simulink model "SF108A_MotCurrPeakEstimn"  (R2013b)
settings: Solver=FixedStepDiscrete  StartTime=0.0  StopTime=1  FixedStep=Ts  RelTol=1e-3
undefined symbols (not defined in the file): ARCHGLBPRM_100MILLISEC_SEC_F32, ARCHGLBPRM_2MILLISEC_SEC_F32
libraries: Fil x6, NxtrLim x2, simulink x1
settings Model: Creator=qzwc4r  LastModifiedBy=BZHF94
settings DataIOCC: LimitDataPoints=off  SaveFormat=Structure  ReturnWorkspaceOutputs=on
settings OptimizationCC: BlockReduction=off  InlineParams=on  ZeroExternalMemoryAtStartup=off  ZeroInternalMemoryAtStartup=off  OptimizeModelRefInitCode=on  LifeSpan=1
settings DebuggingCC: SignalInfNanChecking=error  SignalRangeChecking=warning  UnderspecifiedInitializationDetection=Simplified  SolverPrmCheckMsg=error  InheritedTsInSrcMsg=error  DiscreteInheritContinuousMsg=error  SingleTaskRateTransMsg=error  TasksWithSamePriorityMsg=error  SigSpecEnsureSampleTimeMsg=error  CheckMatrixSingularityMsg=error  IntegerOverflowMsg=error  ParameterUnderflowMsg=error  ParameterPrecisionLossMsg=error  ParameterTunabilityLossMsg=error  FixptConstUnderflowMsg=warning  FixptConstOverflowMsg=warning  VectorMatrixConversionMsg=error  SignalLabelMismatchMsg=error  UnconnectedInputMsg=error  UnconnectedOutputMsg=error  UnconnectedLineMsg=error  SFcnCompatibilityMsg=error  UniqueDataStoreMsg=warning  BusObjectLabelMismatch=error  RootOutportRequireBusObject=error  AssertControl=DisableAll  ModelReferenceIOMsg=error  ModelReferenceVersionMismatchMessage=warning  ModelReferenceIOMismatchMessage=error  ModelReferenceCSMismatchMessage=warning  ModelReferenceDataLoggingMessage=error  StateNameClashWarn=warning  StrictBusMsg=ErrorOnBusTreatedAsVector  NonBusSignalsTreatedAsBus=error  SFUnexpectedBacktrackingDiag=error  SFInvalidInputDataAccessInChartInitDiag=error  SFNoUnconditionalDefaultTransitionDiag=error  SFTransitionOutsideNaturalParentDiag=error  SFUnconditionalTransitionShadowingDiag=error  SFUndirectedBroadcastEventsDiag=error
settings ModelReferenceCC: ModelReferenceNumInstancesAllowed=Single
settings RTWCC: SystemTargetFile=autosar.tlc  GenCodeOnly=on  TemplateMakefile=ert_default_tmf  Description=AUTOSAR  GenerateReport=on  ProcessScript=autosar_make_rtw_hook  LaunchReport=on
settings CodeAppCC: GenerateComments=off  IgnoreCustomStorageClasses=off  CustomSymbolStrType=$N$R$M  CustomSymbolStrBlkIO=$N$M  SimulinkBlockComments=off
settings STFCustomTargetCC: ParMdlRefBuildCompliant=on  CompOptLevelCompliant=on  IncludeMdlTerminateFcn=off  CombineOutputUpdateFcns=on  SuppressErrorStatus=on  ERTFirstTimeCompliant=on  ERTCustomFileBanners=on  SupportNonFinite=off  SupportComplex=off  SupportContinuousTime=off  SupportNonInlinedSFcns=off  MATLABClassNameForMDSCustomization=Simulink.SoftwareTarget.ERTCustomization  AutosarCompliant=on  GRTInterface=off  SystemTargetFile=autosar.tlc
settings ERTTargetCC: CodeReplacementLibrary=ANSI_C  ConcurrentExecutionCompliant=off  IncludeMdlTerminateFcn=off  SuppressErrorStatus=on  SupportNonFinite=off  SupportComplex=off  ModelStepFunctionPrototypeControlCompliant=off  CPPClassGenCompliant=off  AutosarCompliant=on  InlinedParameterPlacement=NonHierarchical  ERTCustomFileTemplate=example_file_process.tlc  EnableUserReplacementTypes=on

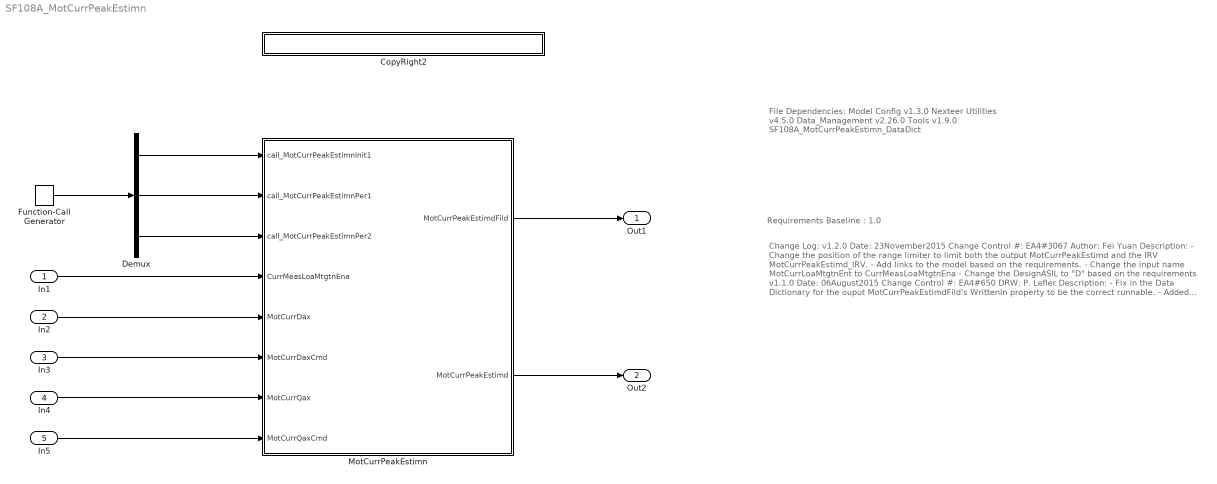
== system SF108A_MotCurrPeakEstimn ==
  note: Requirements Baseline : 1.0
  note: File Dependencies:
      |
      | Model Config v1.3.0
      | Nexteer Utilities v4.5.0
      | Data_Management v2.26.0
      | Tools v1.9.0
      | SF108A_MotCurrPeakEstimn_DataDict
  note: Change Log:
      |
      | v1.2.0
      | Date: 23November2015
      | Change Control #: EA4#3067
      | Author: Fei Yuan
      | Description:
      | - Change the position of the range limiter to limit both the output MotCurrPeakEstimd
      |   and the IRV MotCurrPeakEstimd_IRV.
      | - Add links to the model based on the requirements.
      | - Change the input name MotCurrLoaMtgtnEnt to CurrMeasLoaMtgtnEna
      | - Change the DesignASIL to "D" based on the requirements
      |
      | v1.1.0
      | Date: 06August2015
      | Change Control #: EA4#650
      | DRW: P. Lefler
      | Description:
      | - Fix in the Data Dictionary for the ouput MotCurrPeakEstimdFild's WrittenIn
      |    property to be the correct runnable.
      | - Added range limiters to both of the functions outputs.
      |
      | v1.0.0
      | Date: 17July2015
      | Change Control #: EA4#650
      | DRW: P. Lefler
      | Description:
      | - Initial Release
  In1 : Inport
  In2 : Inport  Port=2
  In3 : Inport  Port=3
  In4 : Inport  Port=4
  In5 : Inport  Port=5
  CopyRight2 : Subsystem  Description=|  mask(Copyright Information){none=on}
      | Copyright info block.                                               
      |                                                                     
      | Place copyright information at the top of every subsystem in design.
      mask prompts: none "No parameters"
      mask help: Place copyright information at the top of every subsystem in design.
      mask Display:
      | NxtrConf = 'Nexteer Confidential';
      | 
      | sys = bdroot; %handle for the current model ("system")
      | first = get_param(sys,'Created');
      | if(isempty(first))
      |     first = datestr(now,'yyyy');
      | else
      |     first = first(end-3:end);  %year is last four digits
      | end
      | 
      | last = get_param(sys,'LastModifiedDate');
      | if isempty(last)
      |     last = datestr(now,'yyyy');
      | else
      |     last = last(end-3:end);
      | end
      | 
      | if strcmp(first,last)
      |     fprintf('%s -- Copyright %s Nexteer',NxtrConf,first)
      | else
      |     fprintf('%s -- %s%s- %s Nexteer',NxtrConf,char(169),first,last)
      | end
  Demux : Demux  Outputs=3
  Function-Call Generator : simulink/Ports & Subsystems/Function-Call Generator  sample_time=0.002  numberOfIterations=1
  MotCurrPeakEstimn : Subsystem
  Out1 : Outport
  Out2 : Outport  Port=2
  wires:
  Demux/3 -> MotCurrPeakEstimn/3(call_MotCurrPeakEstimnPer2)
  Demux/2 -> MotCurrPeakEstimn/2(call_MotCurrPeakEstimnPer1)
  Demux/1 -> MotCurrPeakEstimn/1(call_MotCurrPeakEstimnInit1)
  Function-Call Generator/1 -> Demux/1
  In1/1 -> MotCurrPeakEstimn/4(CurrMeasLoaMtgtnEna)
  In5/1 -> MotCurrPeakEstimn/8(MotCurrQaxCmd)
  In4/1 -> MotCurrPeakEstimn/7(MotCurrQax)
  In3/1 -> MotCurrPeakEstimn/6(MotCurrDaxCmd)
  In2/1 -> MotCurrPeakEstimn/5(MotCurrDax)
  MotCurrPeakEstimn/2(MotCurrPeakEstimd) -> Out2/1
  MotCurrPeakEstimn/1(MotCurrPeakEstimdFild) -> Out1/1

== system SF108A_MotCurrPeakEstimn/CopyRight2 ==

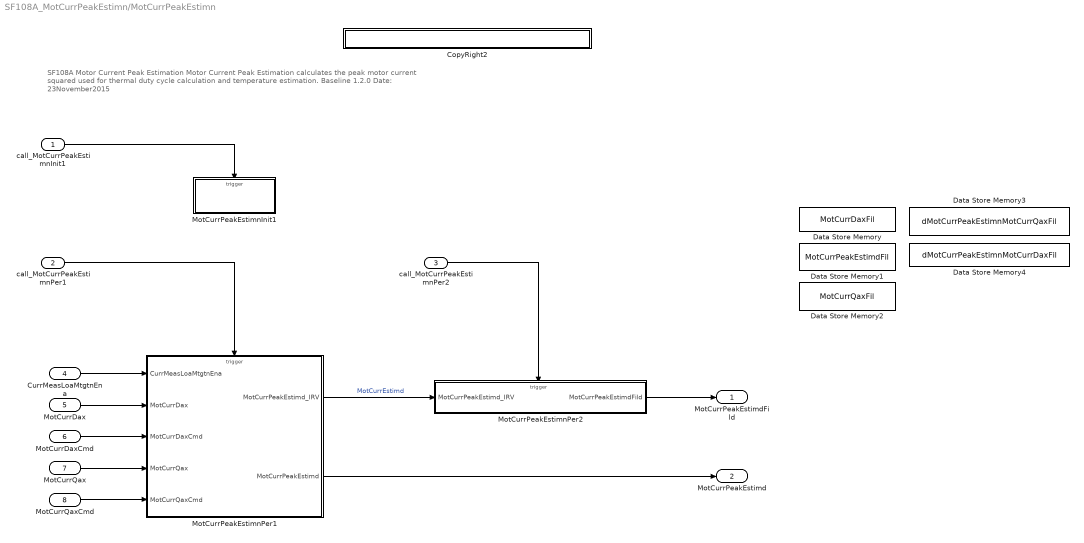
== system SF108A_MotCurrPeakEstimn/MotCurrPeakEstimn ==
  note: SF108A Motor Current Peak Estimation
      | Motor Current Peak Estimation calculates the peak motor current squared used for thermal duty cycle calculation and temperature estimation.
      | Baseline 1.2.0   						Date: 23November2015
  call_MotCurrPeakEstimnInit1 : Inport
  call_MotCurrPeakEstimnPer1 : Inport  RequirementInfo="{'linktype_rmi_doors' '0000bb47 (/E-STEER Core/SubSystem Specifications/Application Functions/SF99/SF108A Motor Peak Current Estimation)' '#SF108A_60' 'true' 'REQ:  SF108A_60' '' } %GIDa_6bf749d1_e317_435f_a199_b983ebcc4e4e"  Port=2
  call_MotCurrPeakEstimnPer2 : Inport  RequirementInfo="{'linktype_rmi_doors' '0000bb47 (/E-STEER Core/SubSystem Specifications/Application Functions/SF99/SF108A Motor Peak Current Estimation)' '#SF108A_61' 'true' 'REQ:  SF108A_61' '' } %GIDa_a8c9eb8f_1548_474e_a89d_794aff322df2"  Port=3
  CurrMeasLoaMtgtnEna : Inport  RequirementInfo="{'linktype_rmi_doors' '0000bb47 (/E-STEER Core/SubSystem Specifications/Application Functions/SF99/SF108A Motor Peak Current Estimation)' '#SF108A_39' 'true' 'REQ:  SF108A_39' '' } %GIDa_5cba7f27_c055_4e0a_88a5_f6c10767b232"  Port=4
  MotCurrDax : Inport  RequirementInfo="{'linktype_rmi_doors' '0000bb47 (/E-STEER Core/SubSystem Specifications/Application Functions/SF99/SF108A Motor Peak Current Estimation)' '#SF108A_64' 'true' 'REQ:  SF108A_64' '' } %GIDa_5e124af2_16d4_47d0_b4c6_a42f73fbe702"  Port=5
  MotCurrDaxCmd : Inport  RequirementInfo="{'linktype_rmi_doors' '0000bb47 (/E-STEER Core/SubSystem Specifications/Application Functions/SF99/SF108A Motor Peak Current Estimation)' '#SF108A_40' 'true' 'REQ:  SF108A_40' '' } %GIDa_8db68579_f68b_4588_ad3f_79d7468913b7"  Port=6
  MotCurrQax : Inport  RequirementInfo="{'linktype_rmi_doors' '0000bb47 (/E-STEER Core/SubSystem Specifications/Application Functions/SF99/SF108A Motor Peak Current Estimation)' '#SF108A_63' 'true' 'REQ:  SF108A_63' '' } %GIDa_22f838d1_2b9f_4a40_8739_b805aada355b"  Port=7
  MotCurrQaxCmd : Inport  RequirementInfo="{'linktype_rmi_doors' '0000bb47 (/E-STEER Core/SubSystem Specifications/Application Functions/SF99/SF108A Motor Peak Current Estimation)' '#SF108A_41' 'true' 'REQ:  SF108A_41' '' } %GIDa_64d93380_d718_45a2_a0da_ab28786a38db"  Port=8
  CopyRight2 : Subsystem  Description=|  mask(Copyright Information){none=on}
      | Copyright info block.                                               
      |                                                                     
      | Place copyright information at the top of every subsystem in design.
      mask prompts: none "No parameters"
      mask help: Place copyright information at the top of every subsystem in design.
      mask Display:
      | NxtrConf = 'Nexteer Confidential';
      | 
      | sys = bdroot; %handle for the current model ("system")
      | first = get_param(sys,'Created');
      | if(isempty(first))
      |     first = datestr(now,'yyyy');
      | else
      |     first = first(end-3:end);  %year is last four digits
      | end
      | 
      | last = get_param(sys,'LastModifiedDate');
      | if isempty(last)
      |     last = datestr(now,'yyyy');
      | else
      |     last = last(end-3:end);
      | end
      | 
      | if strcmp(first,last)
      |     fprintf('%s -- Copyright %s Nexteer',NxtrConf,first)
      | else
      |     fprintf('%s -- %s%s- %s Nexteer',NxtrConf,char(169),first,last)
      | end
  Data Store Memory : DataStoreMemory  DataStoreName=MotCurrDaxFil  InitialValue=[]  StateMustResolveToSignalObject=on
  Data Store Memory1 : DataStoreMemory  DataStoreName=MotCurrPeakEstimdFil  InitialValue=[]  StateMustResolveToSignalObject=on
  Data Store Memory2 : DataStoreMemory  DataStoreName=MotCurrQaxFil  InitialValue=[]  StateMustResolveToSignalObject=on
  Data Store Memory3 : DataStoreMemory  DataStoreName=dMotCurrPeakEstimnMotCurrQaxFil  ReadBeforeWriteMsg=warning  WriteAfterWriteMsg=warning  WriteAfterReadMsg=warning  InitialValue=[]  StateMustResolveToSignalObject=on
  Data Store Memory4 : DataStoreMemory  DataStoreName=dMotCurrPeakEstimnMotCurrDaxFil  ReadBeforeWriteMsg=warning  WriteAfterWriteMsg=warning  WriteAfterReadMsg=warning  InitialValue=[]  StateMustResolveToSignalObject=on
  MotCurrPeakEstimnInit1 : Subsystem
  MotCurrPeakEstimnPer1 : Subsystem
  MotCurrPeakEstimnPer2 : Subsystem
  MotCurrPeakEstimdFild : Outport  RequirementInfo="{'linktype_rmi_doors' '0000bb47 (/E-STEER Core/SubSystem Specifications/Application Functions/SF99/SF108A Motor Peak Current Estimation)' '#SF108A_45' 'true' 'REQ:  SF108A_45' '' } %GIDa_a1170dcc_5009_425a_bdba_f4706c36d75d"
  MotCurrPeakEstimd : Outport  RequirementInfo="{'linktype_rmi_doors' '0000bb47 (/E-STEER Core/SubSystem Specifications/Application Functions/SF99/SF108A Motor Peak Current Estimation)' '#SF108A_42' 'true' 'REQ:  SF108A_42' '' } %GIDa_94c0116b_4fb4_4439_933d_95e745bf3a31"  Port=2
  wires:
  MotCurrDaxCmd/1 -> MotCurrPeakEstimnPer1/3(MotCurrDaxCmd)
  MotCurrQax/1 -> MotCurrPeakEstimnPer1/4(MotCurrQax)
  MotCurrQaxCmd/1 -> MotCurrPeakEstimnPer1/5(MotCurrQaxCmd)
  CurrMeasLoaMtgtnEna/1 -> MotCurrPeakEstimnPer1/1(CurrMeasLoaMtgtnEna)
  MotCurrDax/1 -> MotCurrPeakEstimnPer1/2(MotCurrDax)
  MotCurrPeakEstimnPer1/1(MotCurrPeakEstimd_IRV) -> MotCurrPeakEstimnPer2/1(MotCurrPeakEstimd_IRV)  "MotCurrEstimd"
  MotCurrPeakEstimnPer1/2(MotCurrPeakEstimd) -> MotCurrPeakEstimd/1
  MotCurrPeakEstimnPer2/1(MotCurrPeakEstimdFild) -> MotCurrPeakEstimdFild/1
  call_MotCurrPeakEstimnInit1/1 -> MotCurrPeakEstimnInit1/Trigger
  call_MotCurrPeakEstimnPer1/1 -> MotCurrPeakEstimnPer1/Trigger
  call_MotCurrPeakEstimnPer2/1 -> MotCurrPeakEstimnPer2/Trigger

== system SF108A_MotCurrPeakEstimn/MotCurrPeakEstimn/CopyRight2 ==

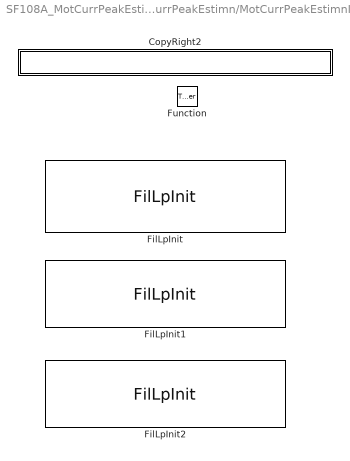
== system SF108A_MotCurrPeakEstimn/MotCurrPeakEstimn/MotCurrPeakEstimnInit1 ==
  Function : TriggerPort  TriggerType=function-call  PortDimensions=1
  CopyRight2 : Subsystem  Description=|  mask(Copyright Information){none=on}
      | Copyright info block.                                               
      |                                                                     
      | Place copyright information at the top of every subsystem in design.
      mask prompts: none "No parameters"
      mask help: Place copyright information at the top of every subsystem in design.
      mask Display:
      | NxtrConf = 'Nexteer Confidential';
      | 
      | sys = bdroot; %handle for the current model ("system")
      | first = get_param(sys,'Created');
      | if(isempty(first))
      |     first = datestr(now,'yyyy');
      | else
      |     first = first(end-3:end);  %year is last four digits
      | end
      | 
      | last = get_param(sys,'LastModifiedDate');
      | if isempty(last)
      |     last = datestr(now,'yyyy');
      | else
      |     last = last(end-3:end);
      | end
      | 
      | if strcmp(first,last)
      |     fprintf('%s -- Copyright %s Nexteer',NxtrConf,first)
      | else
      |     fprintf('%s -- %s%s- %s Nexteer',NxtrConf,char(169),first,last)
      | end
  FilLpInit : Fil/FilLpInit  RequirementInfo="{'linktype_rmi_doors' '0000bb47 (/E-STEER Core/SubSystem Specifications/Application Functions/SF99/SF108A Motor Peak Current Estimation)' '#SF108A_58' 'true' 'REQ:  SF108A_58' '' } %GIDa_e427ef9c_65f9_4120_b498_3b7af46635bb"  Ic=0  Ts=ARCHGLBPRM_100MILLISEC_SEC_F32  Freq=MotCurrPeakEstimnCurrPeakEstimdFilFrq  StVar=MotCurrPeakEstimdFil
  FilLpInit1 : Fil/FilLpInit  RequirementInfo="{'linktype_rmi_doors' '0000bb47 (/E-STEER Core/SubSystem Specifications/Application Functions/SF99/SF108A Motor Peak Current Estimation)' '#SF108A_55' 'true' 'REQ:  SF108A_55' '' ; 'linktype_rmi_doors' '0000bb47 (/E-STEER Core/SubSystem Specifications/Application Functions/SF99/SF108A Motor Peak Current Estimation)' '#SF108A_54' 'true' 'REQ:  SF108A_54' '' } %GIDa_b3aebcc8_791a_48c6_871c_fe27388f4f19"  Ic=0  Ts=ARCHGLBPRM_2MILLISEC_SEC_F32  Freq=MotCurrPeakEstimnCurrFilFrq  StVar=MotCurrDaxFil
  FilLpInit2 : Fil/FilLpInit  RequirementInfo="{'linktype_rmi_doors' '0000bb47 (/E-STEER Core/SubSystem Specifications/Application Functions/SF99/SF108A Motor Peak Current Estimation)' '#SF108A_53' 'true' 'REQ:  SF108A_53' '' ; 'linktype_rmi_doors' '0000bb47 (/E-STEER Core/SubSystem Specifications/Application Functions/SF99/SF108A Motor Peak Current Estimation)' '#SF108A_51' 'true' 'REQ:  SF108A_51' '' } %GIDa_9d23ef10_2f40_4bd1_a4f3_61fe2efc73b8"  Ic=0  Ts=ARCHGLBPRM_2MILLISEC_SEC_F32  Freq=MotCurrPeakEstimnCurrFilFrq  StVar=MotCurrQaxFil

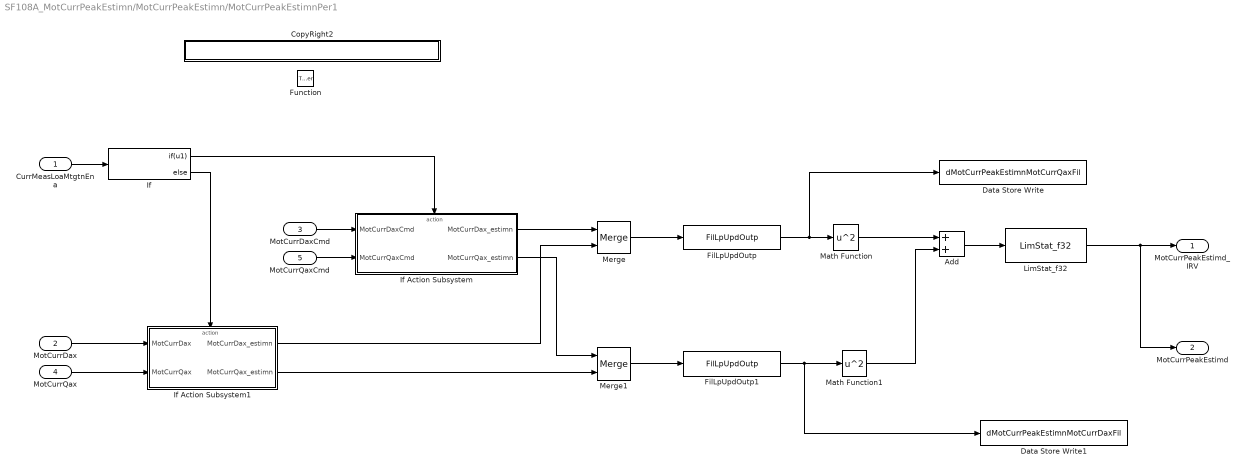
== system SF108A_MotCurrPeakEstimn/MotCurrPeakEstimn/MotCurrPeakEstimnPer1 ==
  CurrMeasLoaMtgtnEna : Inport
  MotCurrDax : Inport  Port=2
  MotCurrDaxCmd : Inport  Port=3
  MotCurrQax : Inport  Port=4
  MotCurrQaxCmd : Inport  Port=5
  Function : TriggerPort  TriggerType=function-call  PortDimensions=1
  Add : Sum  RequirementInfo="{'linktype_rmi_doors' '0000bb47 (/E-STEER Core/SubSystem Specifications/Application Functions/SF99/SF108A Motor Peak Current Estimation)' '#SF108A_56' 'true' 'REQ:  SF108A_56' '' } %GIDa_0d214596_a876_4096_94d5_b9558133ccfd"
  CopyRight2 : Subsystem  Description=|  mask(Copyright Information){none=on}
      | Copyright info block.                                               
      |                                                                     
      | Place copyright information at the top of every subsystem in design.
      mask prompts: none "No parameters"
      mask help: Place copyright information at the top of every subsystem in design.
      mask Display:
      | NxtrConf = 'Nexteer Confidential';
      | 
      | sys = bdroot; %handle for the current model ("system")
      | first = get_param(sys,'Created');
      | if(isempty(first))
      |     first = datestr(now,'yyyy');
      | else
      |     first = first(end-3:end);  %year is last four digits
      | end
      | 
      | last = get_param(sys,'LastModifiedDate');
      | if isempty(last)
      |     last = datestr(now,'yyyy');
      | else
      |     last = last(end-3:end);
      | end
      | 
      | if strcmp(first,last)
      |     fprintf('%s -- Copyright %s Nexteer',NxtrConf,first)
      | else
      |     fprintf('%s -- %s%s- %s Nexteer',NxtrConf,char(169),first,last)
      | end
  Data Store Write : DataStoreWrite  DataStoreName=dMotCurrPeakEstimnMotCurrQaxFil
  Data Store Write1 : DataStoreWrite  DataStoreName=dMotCurrPeakEstimnMotCurrDaxFil
  FilLpUpdOutp : Fil/FilLpUpdOutp  RequirementInfo="{'linktype_rmi_doors' '0000bb47 (/E-STEER Core/SubSystem Specifications/Application Functions/SF99/SF108A Motor Peak Current Estimation)' '#SF108A_51' 'true' 'REQ:  SF108A_51' '' } %GIDa_b1d70a8a_d6cc_4e94_a1d9_7601c375e32a"  StVar=MotCurrDaxFil
      settings: AttributesFormatString=StVar: %<StVar>
  FilLpUpdOutp1 : Fil/FilLpUpdOutp  RequirementInfo="{'linktype_rmi_doors' '0000bb47 (/E-STEER Core/SubSystem Specifications/Application Functions/SF99/SF108A Motor Peak Current Estimation)' '#SF108A_51' 'true' 'REQ:  SF108A_51' '' } %GIDa_fb2a96c2_20a1_4e11_95e0_4988bdcb45e1"  StVar=MotCurrQaxFil
      settings: AttributesFormatString=StVar: %<StVar>
  If : If  RequirementInfo="{'linktype_rmi_doors' '0000bb47 (/E-STEER Core/SubSystem Specifications/Application Functions/SF99/SF108A Motor Peak Current Estimation)' '#SF108A_48' 'true' 'REQ:  SF108A_48' '' ; 'linktype_rmi_doors' '0000bb47 (/E-STEER Core/SubSystem Specifications/Application Functions/SF99/SF108A Motor Peak Current Estimation)' '#SF108A_49' 'true' 'REQ:  SF108A_49' '' } %GIDa_bbfe8313_fdca_4091_8257_8aa98929a7c3"  IfExpression=u1
  If Action Subsystem : Subsystem  RequirementInfo="{'linktype_rmi_doors' '0000bb47 (/E-STEER Core/SubSystem Specifications/Application Functions/SF99/SF108A Motor Peak Current Estimation)' '#SF108A_48' 'true' 'REQ:  SF108A_48' '' ; 'linktype_rmi_doors' '0000bb47 (/E-STEER Core/SubSystem Specifications/Application Functions/SF99/SF108A Motor Peak Current Estimation)' '#SF108A_49' 'true' 'REQ:  SF108A_49' '' } %GIDa_01cb091a_0ed1_4490_8550_d6d7aca05513"  TreatAsAtomicUnit=on
  If Action Subsystem1 : Subsystem  RequirementInfo="{'linktype_rmi_doors' '0000bb47 (/E-STEER Core/SubSystem Specifications/Application Functions/SF99/SF108A Motor Peak Current Estimation)' '#SF108A_48' 'true' 'REQ:  SF108A_48' '' ; 'linktype_rmi_doors' '0000bb47 (/E-STEER Core/SubSystem Specifications/Application Functions/SF99/SF108A Motor Peak Current Estimation)' '#SF108A_49' 'true' 'REQ:  SF108A_49' '' } %GIDa_65cb279a_aed7_4015_b668_f3189407b7cd"  TreatAsAtomicUnit=on
  LimStat_f32 : NxtrLim/LimStat_f32  RequirementInfo="{'linktype_rmi_doors' '0000bb47 (/E-STEER Core/SubSystem Specifications/Application Functions/SF99/SF108A Motor Peak Current Estimation)' '#SF108A_68' 'true' 'REQ:  SF108A_68' '' } %GIDa_6cd9cc1f_6b05_4da1_ae59_10dd91c732d6"  LoLim=MOTCURRPEAKMIN_AMPRSQD_F32  HiLim=MOTCURRPEAKMAX_AMPRSQD_F32
      settings: AttributesFormatString=|
      | Low Limit: %<LoLim>
      | High Limit:%<HiLim>
  Math Function : Math  RequirementInfo="{'linktype_rmi_doors' '0000bb47 (/E-STEER Core/SubSystem Specifications/Application Functions/SF99/SF108A Motor Peak Current Estimation)' '#SF108A_56' 'true' 'REQ:  SF108A_56' '' } %GIDa_98b5c497_9b69_4612_930a_769c70e2bf53"  Operator=square  SaturateOnIntegerOverflow=on
  Math Function1 : Math  RequirementInfo="{'linktype_rmi_doors' '0000bb47 (/E-STEER Core/SubSystem Specifications/Application Functions/SF99/SF108A Motor Peak Current Estimation)' '#SF108A_56' 'true' 'REQ:  SF108A_56' '' } %GIDa_1bc240d6_1e82_4846_b18b_2ce4df9d92b7"  Operator=square  SaturateOnIntegerOverflow=on
  Merge : Merge  RequirementInfo="{'linktype_rmi_doors' '0000bb47 (/E-STEER Core/SubSystem Specifications/Application Functions/SF99/SF108A Motor Peak Current Estimation)' '#SF108A_48' 'true' 'REQ:  SF108A_48' '' ; 'linktype_rmi_doors' '0000bb47 (/E-STEER Core/SubSystem Specifications/Application Functions/SF99/SF108A Motor Peak Current Estimation)' '#SF108A_49' 'true' 'REQ:  SF108A_49' '' } %GIDa_0a276253_a3e1_4688_8311_e5e3668e937a"
  Merge1 : Merge  RequirementInfo="{'linktype_rmi_doors' '0000bb47 (/E-STEER Core/SubSystem Specifications/Application Functions/SF99/SF108A Motor Peak Current Estimation)' '#SF108A_48' 'true' 'REQ:  SF108A_48' '' ; 'linktype_rmi_doors' '0000bb47 (/E-STEER Core/SubSystem Specifications/Application Functions/SF99/SF108A Motor Peak Current Estimation)' '#SF108A_49' 'true' 'REQ:  SF108A_49' '' } %GIDa_20ef0638_b181_477f_8f20_5b87fcc2f56e"
  MotCurrPeakEstimd_IRV : Outport
  MotCurrPeakEstimd : Outport  Port=2
  wires:
  If/1 -> If Action Subsystem/Action
  If/2 -> If Action Subsystem1/Action
  MotCurrDaxCmd/1 -> If Action Subsystem/1(MotCurrDaxCmd)
  MotCurrQaxCmd/1 -> If Action Subsystem/2(MotCurrQaxCmd)
  MotCurrDax/1 -> If Action Subsystem1/1(MotCurrDax)
  MotCurrQax/1 -> If Action Subsystem1/2(MotCurrQax)
  If Action Subsystem/1(MotCurrDax_estimn) -> Merge/1
  If Action Subsystem1/1(MotCurrDax_estimn) -> Merge/2
  If Action Subsystem/2(MotCurrQax_estimn) -> Merge1/1
  If Action Subsystem1/2(MotCurrQax_estimn) -> Merge1/2
  Merge/1 -> FilLpUpdOutp/1
  Merge1/1 -> FilLpUpdOutp1/1
  FilLpUpdOutp/1 -> Data Store Write/1, Math Function/1
  Math Function/1 -> Add/1
  Math Function1/1 -> Add/2
  CurrMeasLoaMtgtnEna/1 -> If/1
  FilLpUpdOutp1/1 -> Data Store Write1/1, Math Function1/1
  Add/1 -> LimStat_f32/1
  LimStat_f32/1 -> MotCurrPeakEstimd/1, MotCurrPeakEstimd_IRV/1

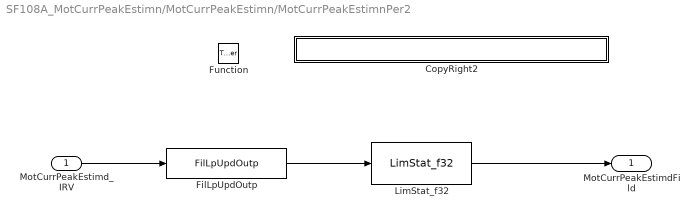
== system SF108A_MotCurrPeakEstimn/MotCurrPeakEstimn/MotCurrPeakEstimnPer2 ==
  MotCurrPeakEstimd_IRV : Inport
  Function : TriggerPort  TriggerType=function-call  PortDimensions=1
  CopyRight2 : Subsystem  Description=|  mask(Copyright Information){none=on}
      | Copyright info block.                                               
      |                                                                     
      | Place copyright information at the top of every subsystem in design.
      mask prompts: none "No parameters"
      mask help: Place copyright information at the top of every subsystem in design.
      mask Display:
      | NxtrConf = 'Nexteer Confidential';
      | 
      | sys = bdroot; %handle for the current model ("system")
      | first = get_param(sys,'Created');
      | if(isempty(first))
      |     first = datestr(now,'yyyy');
      | else
      |     first = first(end-3:end);  %year is last four digits
      | end
      | 
      | last = get_param(sys,'LastModifiedDate');
      | if isempty(last)
      |     last = datestr(now,'yyyy');
      | else
      |     last = last(end-3:end);
      | end
      | 
      | if strcmp(first,last)
      |     fprintf('%s -- Copyright %s Nexteer',NxtrConf,first)
      | else
      |     fprintf('%s -- %s%s- %s Nexteer',NxtrConf,char(169),first,last)
      | end
  FilLpUpdOutp : Fil/FilLpUpdOutp  RequirementInfo="{'linktype_rmi_doors' '0000bb47 (/E-STEER Core/SubSystem Specifications/Application Functions/SF99/SF108A Motor Peak Current Estimation)' '#SF108A_58' 'true' 'REQ:  SF108A_58' '' } %GIDa_dcfc624a_2036_4b55_8c20_164b1f7e99f4"  StVar=MotCurrPeakEstimdFil
      settings: AttributesFormatString=StVar: %<StVar>
  LimStat_f32 : NxtrLim/LimStat_f32  RequirementInfo="{'linktype_rmi_doors' '0000bb47 (/E-STEER Core/SubSystem Specifications/Application Functions/SF99/SF108A Motor Peak Current Estimation)' '#SF108A_68' 'true' 'REQ:  SF108A_68' '' } %GIDa_56246546_97af_4fdd_aa23_1038f1a855fb"  LoLim=MOTCURRPEAKMIN_AMPRSQD_F32  HiLim=MOTCURRPEAKMAX_AMPRSQD_F32
      settings: AttributesFormatString=|
      | Low Limit: %<LoLim>
      | High Limit:%<HiLim>
  MotCurrPeakEstimdFild : Outport
  wires:
  FilLpUpdOutp/1 -> LimStat_f32/1
  MotCurrPeakEstimd_IRV/1 -> FilLpUpdOutp/1
  LimStat_f32/1 -> MotCurrPeakEstimdFild/1

== system SF108A_MotCurrPeakEstimn/MotCurrPeakEstimn/MotCurrPeakEstimnInit1/CopyRight2 ==

== system SF108A_MotCurrPeakEstimn/MotCurrPeakEstimn/MotCurrPeakEstimnPer1/CopyRight2 ==

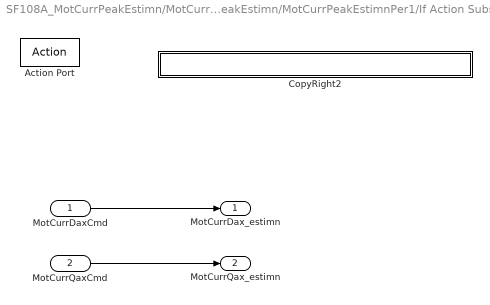
== system SF108A_MotCurrPeakEstimn/MotCurrPeakEstimn/MotCurrPeakEstimnPer1/If Action Subsystem ==
  MotCurrDaxCmd : Inport
  MotCurrQaxCmd : Inport  Port=2
  Action Port : ActionPort  ActionType=then
  CopyRight2 : Subsystem  Description=|  mask(Copyright Information){none=on}
      | Copyright info block.                                               
      |                                                                     
      | Place copyright information at the top of every subsystem in design.
      mask prompts: none "No parameters"
      mask help: Place copyright information at the top of every subsystem in design.
      mask Display:
      | NxtrConf = 'Nexteer Confidential';
      | 
      | sys = bdroot; %handle for the current model ("system")
      | first = get_param(sys,'Created');
      | if(isempty(first))
      |     first = datestr(now,'yyyy');
      | else
      |     first = first(end-3:end);  %year is last four digits
      | end
      | 
      | last = get_param(sys,'LastModifiedDate');
      | if isempty(last)
      |     last = datestr(now,'yyyy');
      | else
      |     last = last(end-3:end);
      | end
      | 
      | if strcmp(first,last)
      |     fprintf('%s -- Copyright %s Nexteer',NxtrConf,first)
      | else
      |     fprintf('%s -- %s%s- %s Nexteer',NxtrConf,char(169),first,last)
      | end
  MotCurrDax_estimn : Outport
  MotCurrQax_estimn : Outport  Port=2
  wires:
  MotCurrDaxCmd/1 -> MotCurrDax_estimn/1
  MotCurrQaxCmd/1 -> MotCurrQax_estimn/1

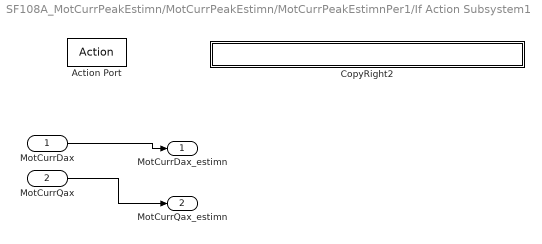
== system SF108A_MotCurrPeakEstimn/MotCurrPeakEstimn/MotCurrPeakEstimnPer1/If Action Subsystem1 ==
  MotCurrDax : Inport
  MotCurrQax : Inport  Port=2
  Action Port : ActionPort  ActionType=else
  CopyRight2 : Subsystem  Description=|  mask(Copyright Information){none=on}
      | Copyright info block.                                               
      |                                                                     
      | Place copyright information at the top of every subsystem in design.
      mask prompts: none "No parameters"
      mask help: Place copyright information at the top of every subsystem in design.
      mask Display:
      | NxtrConf = 'Nexteer Confidential';
      | 
      | sys = bdroot; %handle for the current model ("system")
      | first = get_param(sys,'Created');
      | if(isempty(first))
      |     first = datestr(now,'yyyy');
      | else
      |     first = first(end-3:end);  %year is last four digits
      | end
      | 
      | last = get_param(sys,'LastModifiedDate');
      | if isempty(last)
      |     last = datestr(now,'yyyy');
      | else
      |     last = last(end-3:end);
      | end
      | 
      | if strcmp(first,last)
      |     fprintf('%s -- Copyright %s Nexteer',NxtrConf,first)
      | else
      |     fprintf('%s -- %s%s- %s Nexteer',NxtrConf,char(169),first,last)
      | end
  MotCurrDax_estimn : Outport
  MotCurrQax_estimn : Outport  Port=2
  wires:
  MotCurrDax/1 -> MotCurrDax_estimn/1
  MotCurrQax/1 -> MotCurrQax_estimn/1

== system SF108A_MotCurrPeakEstimn/MotCurrPeakEstimn/MotCurrPeakEstimnPer2/CopyRight2 ==

== system SF108A_MotCurrPeakEstimn/MotCurrPeakEstimn/MotCurrPeakEstimnPer1/If Action Subsystem/CopyRight2 ==

== system SF108A_MotCurrPeakEstimn/MotCurrPeakEstimn/MotCurrPeakEstimnPer1/If Action Subsystem1/CopyRight2 ==
